simulink model "task_2_scheme"  (R2024a)
settings: Solver=FixedStepAuto  StartTime=0.0  StopTime=3.0  FixedStep=1e-3  RelTol=1e-6
settings Model: Creator=alexe  LastModifiedBy=alexe

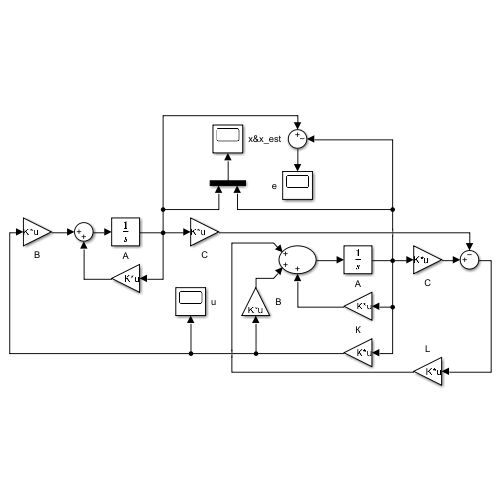
[thumbnail: Simulink's stored preview of the top-level diagram]
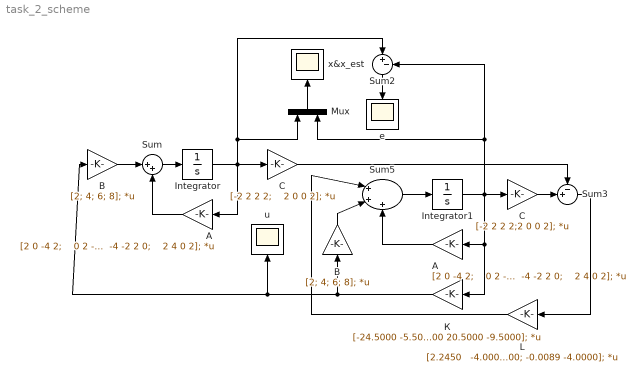
== system task_2_scheme ==
  A : Gain  Gain=|  Multiplication=Matrix(K*u)
      | [2 0 -4 2;
      |    0 2 -2 4;
      |   -4 -2 2 0;
      |    2 4 0 2];
  B : Gain  Gain=[2; 4; 6; 8];  Multiplication=Matrix(K*u)
  C : Gain  Gain=|  Multiplication=Matrix(K*u)
      | [-2 2 2 2;
      |    2 0 0 2];
  Integrator : Integrator  InitialCondition=[1;1;1;1]
  Integrator1 : Integrator  InitialCondition=[0; 0; 0; 0]
  L : Gain  Gain=|  Multiplication=Matrix(K*u)
      | [2.2450   -4.0000; -0.1281 -8.0000; -2.1222 8.0000;
      | -0.0089 -4.0000];
  Mux : Mux  Inputs=2
  Sum : Sum  Inputs=|++
  Sum2 : Sum  Inputs=|+-
  Sum3 : Sum  Inputs=-+|
  Sum5 : Sum  Inputs=|+++
  e : Scope
  u : Scope
  x&x_est : Scope
  А : Gain  Gain=|  Multiplication=Matrix(K*u)
      | [2 0 -4 2;
      |    0 2 -2 4;
      |   -4 -2 2 0;
      |    2 4 0 2];
  В : Gain  Gain=[2; 4; 6; 8];  Multiplication=Matrix(K*u)
  К : Gain  Gain=[-24.5000 -5.5000 20.5000 -9.5000];  Multiplication=Matrix(K*u)
  С : Gain  Gain=[-2 2 2 2;2 0 0 2];  Multiplication=Matrix(K*u)
  wires:
  B/1 -> Sum/1
  Sum/1 -> Integrator/1
  A/1 -> Sum/2
  Integrator/1 -> Sum2/1, Mux/1, C/1, A/1
  К/1 -> B/1, u/1, В/1
  Mux/1 -> x&x_est/1
  Sum2/1 -> e/1
  Integrator1/1 -> Sum2/2, Mux/2, К/1, А/1, С/1
  С/1 -> Sum3/2
  C/1 -> Sum3/1
  Sum3/1 -> L/1
  Sum5/1 -> Integrator1/1
  А/1 -> Sum5/3
  L/1 -> Sum5/1
  В/1 -> Sum5/2
